simulink library "xpcnilib"  (Simulink 6.0)
settings: Solver=ode45  SolverMode=SingleTasking  StartTime=0.0  StopTime=10.0  RelTol=1e-3
undefined symbols (not defined in the file or in its folder): madnipcie, mctrnipcie, mctrnipciecap, mdacbisa, mdanipci670x, mdanipci671x, mdanipcie, mdionipci6527, mdionipcie, mencnipci660x, misa8255, mnigpib, mnipci660x, mpci8255
libraries: xpcmeasurementcomputinglib x6
(part 3 of 3)

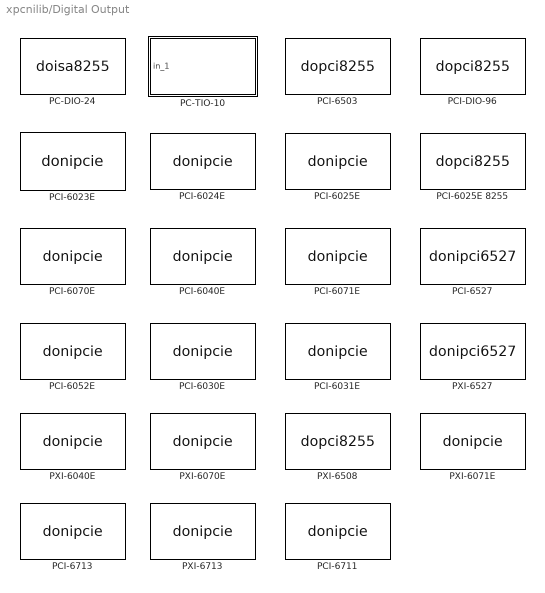
== system xpcnilib/Digital Output ==
  "PC-DIO-24 " : S-Function  InitFcn=misa8255(1);  FunctionName=doisa8255  Parameters=channel, port, reset, initValue, sampletime, baseaddress, control  mask(donipcdio24){channel=[1], port=A, reset=[1], initValue=[0], chip=1, sampletime=0.001, baseaddress=0x300}
      mask prompts: channel "Channel vector:"; reset "Reset vector:"; initValue "Initial value vector:"; sampletime "Sample time:"; baseaddress "Base address (i.e. 0xd000):"
      mask help:
      | PC-DIO-24
      | National Instruments
      | Digital Output
      mask init:
      | baseaddress=hex2dec(baseaddress(3:end));
      | control=155;
      | boardType=16;
      | [baseaddress,control,maskdisplay,maskdescription,reset,initValue]=misa8255(2, chip, port, channel, baseaddress, reset, initValue);
      | set_param(gcb, 'MaskDisplay', maskdisplay);
      | set_param(gcb, 'MaskDescription', maskdescription);
      mask Help: helpview(fullfile(docroot, 'mapfiles', 'xpc.map'), 'NationalInstruments_PC-DIO-24_DOUT')
      mask StyleString: edit,popup(A|B|C),edit,edit,popup(1),edit,edit
      mask Display: disp('PC-DIO-24\nNational Instr.\nDigital Output');port_label('input',1,'1');
  "PC-TIO-10 " : Subsystem  PropExecContextAcrossSSBoundary=on  mask(Digital Output Module){n_channels=1, port=PIA A, sample_time=0.001, baseaddress=0x300}
      mask prompts: n_channels "Number of channels:"; sample_time "Sample time:"; baseaddress "Base address (i.e. 0xd000):"
      mask help:
      | PC-TIO-10
      | National Instruments
      | Digital Output
      mask init:
      | baseaddress=hex2dec(baseaddress(3:end));
      mask Help: helpview(fullfile(docroot, 'mapfiles', 'xpc.map'), 'NationalInstruments_PC-TIO-10_DOUT')
      mask StyleString: edit,popup(PIA A|PIA B),edit,edit
      mask Display: disp('PC-TIO-10\nNational Instr.\nDigital Output')
  "PCI-6023E " : S-Function  InitFcn=mdionipcie(1);  FunctionName=donipcie  Parameters="channel,  reset, initValue, sampletime,slot, control, boardType"  mask(donipcie){channel=[1], reset=[1], initValue=[0], sampletime=0.001, slot=-1}
      mask prompts: channel "Channel vector:"; reset "Reset vector:"; initValue "Initial value vector:"; sampletime "Sample time:"; slot "PCI slot (-1: autosearch):"
      mask help:
      | PCI-6023E
      | National Instruments
      | Digital Output
      mask init:
      | control=0;
      | boardType=1;
      | [control,reset,initValue]=mdionipcie(2,channel,slot,2,boardType,reset,initValue);
      mask Help: helpview(fullfile(docroot, 'mapfiles', 'xpc.map'), 'NationalInstruments_PCI-6023E_DOUT')
      mask Display: disp('PCI-6023E\nNational Instr.\nDigital Output');port_label('input',1,'1');
  "PCI-6024E " : S-Function  InitFcn=mdionipcie(1);  FunctionName=donipcie  Parameters=channel, reset, initValue, sampletime,slot, control, boardType  mask(donipcie){channel=[1], reset=[1], initValue=[0], sampletime=0.001, slot=-1}
      mask prompts: channel "Channel vector:"; reset "Reset vector:"; initValue "Initial value vector:"; sampletime "Sample time:"; slot "PCI slot (-1: autosearch):"
      mask help:
      | PCI-6024E
      | National Instruments
      | Digital Output
      mask init:
      | control=0;
      | boardType=2;
      | [control,reset,initValue]=mdionipcie(2,channel,slot,2,boardType,reset,initValue);
      mask Help: helpview(fullfile(docroot, 'mapfiles', 'xpc.map'), 'NationalInstruments_PCI-6024E_DOUT')
      mask Display: disp('PCI-6024E\nNational Instr.\nDigital Output');port_label('input',1,'1');
  "PCI-6025E " : S-Function  InitFcn=mdionipcie(1);  FunctionName=donipcie  Parameters=channel, reset, initValue, sampletime,slot, control, boardType  mask(donipcie){channel=[1], reset=[1], initValue=[0], sampletime=0.001, slot=-1}
      mask prompts: channel "Channel vector:"; reset "Reset vector:"; initValue "Initial value vector:"; sampletime "Sample time:"; slot "PCI slot (-1: autosearch):"
      mask help:
      | PCI-6025E
      | National Instruments
      | Digital Output
      mask init:
      | control=0;
      | boardType=3;
      | [control,reset,initValue]=mdionipcie(2,channel,slot,2,boardType,reset,initValue);
      mask Help: helpview(fullfile(docroot, 'mapfiles', 'xpc.map'), 'NationalInstruments_PCI-6025E_DOUT')
      mask Display: disp('PCI-6025E\nNational Instr.\nDigital Output');port_label('input',1,'1');
  "PCI-6025E 8255 " : S-Function  InitFcn=mpci8255(1);  FunctionName=dopci8255  Parameters=channel, port, reset, initValue, chip, sampletime, slot, control, boardType  mask(donipci6025e8255){channel=[1], port=A, reset=[1], initValue=[0], chip=1, sampletime=0.001, slot=-1}
      mask prompts: channel "Channel vector:"; reset "Reset vector:"; initValue "Initial value vector:"; sampletime "Sample time:"; slot "PCI slot (-1: autosearch):"
      mask help:
      | PCI-6025E (8255)
      | National Instruments
      | Digital Output
      mask init:
      | control=155;
      | [boardType,control,maskdisplay,maskdescription, reset, initValue]=mpci8255(2, chip, port, channel, slot, reset, initValue);
      | set_param(gcb, 'MaskDisplay', maskdisplay);
      | set_param(gcb, 'MaskDescription', maskdescription);
      mask Help: helpview(fullfile(docroot, 'mapfiles', 'xpc.map'), 'NationalInstruments_PCI-6025E-8255_DOUT')
      mask StyleString: edit,popup(A|B|C),edit,edit,popup(1),edit,edit
      mask Display: disp('PCI-6025E (8255)\nNational Instr.\nDigital Output');port_label('input',1,'1');
  "PCI-6030E " : S-Function  InitFcn=mdionipcie(1);  FunctionName=donipcie  Parameters=channel, reset, initValue, sampletime,slot, control, boardType  mask(donipcie){channel=[1], reset=[1], initValue=[0], sampletime=0.001, slot=-1}
      mask prompts: channel "Channel vector:"; reset "Reset vector:"; initValue "Initial value vector:"; sampletime "Sample time:"; slot "PCI slot (-1: autosearch):"
      mask help:
      | PCI-6030E
      | National Instruments
      | Digital Output
      mask init:
      | control=0;
      | boardType=10;
      | [control,reset,initValue]=mdionipcie(2,channel,slot,2,boardType,reset,initValue);
      mask Help: helpview(fullfile(docroot, 'mapfiles', 'xpc.map'), 'NationalInstruments_PCI-MIO-16XE-10_DOUT')
      mask Display: disp('PCI-6030E\nNational Instr.\nDigital Output');port_label('input',1,'1');
  "PCI-6031E " : S-Function  InitFcn=mdionipcie(1);  FunctionName=donipcie  Parameters=channel, reset, initValue, sampletime,slot, control, boardType  mask(donipcie){channel=[1], reset=[1], initValue=[0], sampletime=0.001, slot=-1}
      mask prompts: channel "Channel vector:"; reset "Reset vector:"; initValue "Initial value vector:"; sampletime "Sample time:"; slot "PCI slot (-1: autosearch):"
      mask help:
      | PCI-6031E
      | National Instruments
      | Digital Output
      mask init:
      | control=0;
      | boardType=11;
      | [control,reset,initValue]=mdionipcie(2,channel,slot,2,boardType,reset,initValue);
      mask Help: helpview(fullfile(docroot, 'mapfiles', 'xpc.map'), 'NationalInstruments_PCI-6031E_DOUT')
      mask Display: disp('PCI-6031E\nNational Instr.\nDigital Output');port_label('input',1,'1');
  "PCI-6040E " : S-Function  InitFcn=mdionipcie(1);  FunctionName=donipcie  Parameters=channel, reset, initValue, sampletime,slot, control, boardType  mask(donipcie){channel=[1], reset=[1], initValue=[0], sampletime=0.001, slot=-1}
      mask prompts: channel "Channel vector:"; reset "Reset vector:"; initValue "Initial value vector:"; sampletime "Sample time:"; slot "PCI slot (-1: autosearch):"
      mask help:
      | PCI-6040E
      | National Instruments
      | Digital Output
      mask init:
      | control=0;
      | boardType=5;
      | [control,reset,initValue]=mdionipcie(2,channel,slot,2,boardType,reset,initValue);
      mask Help: helpview(fullfile(docroot, 'mapfiles', 'xpc.map'), 'NationalInstruments_PCI-MIO-16E-4_DOUT')
      mask Display: disp('PCI-6040E\nNational Instr.\nDigital Output');port_label('input',1,'1');
  "PCI-6052E " : S-Function  InitFcn=mdionipcie(1);  FunctionName=donipcie  Parameters=channel, reset, initValue, sampletime,slot, control, boardType  mask(donipcie){channel=[1], reset=[1], initValue=[0], sampletime=0.001, slot=-1}
      mask prompts: channel "Channel vector:"; reset "Reset vector:"; initValue "Initial value vector:"; sampletime "Sample time:"; slot "PCI slot (-1: autosearch):"
      mask help:
      | PCI-6052E
      | National Instruments
      | Digital Output
      mask init:
      | control=0;
      | boardType=9;
      | [control,reset,initValue]=mdionipcie(2,channel,slot,2,boardType,reset,initValue);
      mask Help: helpview(fullfile(docroot, 'mapfiles', 'xpc.map'), 'NationalInstruments_PCI-6052E_DOUT')
      mask Display: disp('PCI-6052E\nNational Instr.\nDigital Output');port_label('input',1,'1');
  "PCI-6070E " : S-Function  InitFcn=mdionipcie(1);  FunctionName=donipcie  Parameters=channel, reset, initValue, sampletime,slot, control, boardType  mask(donipcie){channel=[1], reset=[1], initValue=[0], sampletime=0.001, slot=-1}
      mask prompts: channel "Channel vector:"; reset "Reset vector:"; initValue "Initial value vector:"; sampletime "Sample time:"; slot "PCI slot (-1: autosearch):"
      mask help:
      | PCI-6070E
      | National Instruments
      | Digital Output
      mask init:
      | control=0;
      | boardType=4;
      | [control,reset,initValue]=mdionipcie(2,channel,slot,2,boardType,reset,initValue);
      mask Help: helpview(fullfile(docroot, 'mapfiles', 'xpc.map'), 'NationalInstruments_PCI-MIO-16E-1_DOUT')
      mask Display: disp('PCI-6070E\nNational Instr.\nDigital Output');port_label('input',1,'1');
  "PCI-6071E " : S-Function  InitFcn=mdionipcie(1);  FunctionName=donipcie  Parameters=channel, reset, initValue, sampletime,slot, control, boardType  mask(donipcie){channel=[1], reset=[1], initValue=[0], sampletime=0.001, slot=-1}
      mask prompts: channel "Channel vector:"; reset "Reset vector:"; initValue "Inital value vector:"; sampletime "Sample time:"; slot "PCI slot (-1: autosearch):"
      mask help:
      | PCI-6071E
      | National Instruments
      | Digital Output
      mask init:
      | control=0;
      | boardType=8;
      | [control,reset,initValue]=mdionipcie(2,channel,slot,2,boardType,reset,initValue);
      mask Help: helpview(fullfile(docroot, 'mapfiles', 'xpc.map'), 'NationalInstruments_PCI-6071E_DOUT')
      mask Display: disp('PCI-6071E\nNational Instr.\nDigital Output');port_label('input',1,'1');
  "PCI-6503 " : S-Function  InitFcn=mpci8255(1);  FunctionName=dopci8255  Parameters=channel, port, reset, initValue, chip, sampletime, slot, control, boardType  mask(donipci6503){channel=[1], port=A, reset=[1], initValue=[0], chip=1, sampletime=0.001, slot=-1}
      mask prompts: channel "Channel vector:"; reset "Reset vector:"; initValue "Initial value vector:"; sampletime "Sample time:"; slot "PCI slot (-1: autosearch):"
      mask help:
      | PCI-6503
      | National Instruments
      | Digital Output
      mask init: same as xpcnilib/Digital Output/PCI-6025E 8255 
      mask Help: helpview(fullfile(docroot, 'mapfiles', 'xpc.map'), 'NationalInstruments_PCI-6503_DOUT')
      mask StyleString: edit,popup(A|B|C),edit,edit,popup(1),edit,edit
      mask Display: disp('PCI-6503\nNational Instr.\nDigital Output');port_label('input',1,'1');
  "PCI-6527 " : S-Function  InitFcn=mdionipci6527(1);  FunctionName=donipci6527  Parameters=channel, port, reset, initValue, sample, slot,1  mask(donipci6527){channel=[1], port=A, reset=[1], initValue=[0], sample=0.001, slot=-1}
      mask prompts: channel "Channel vector:"; reset "Reset vector:"; initValue "Initial value vector:"; sample "Sample time:"; slot "PCI slot (-1: autosearch):"
      mask help:
      | PCI-6527
      | National Instruments
      | Digital Output
      mask init:
      | [filter, reset, initValue] = mdionipci6527( 2, channel, port, sample, slot, 2, 0, 0, reset, initValue );
      mask Help: helpview(fullfile(docroot, 'mapfiles', 'xpc.map'), 'NationalInstruments_PCI-6527_DOUT')
      mask StyleString: edit,popup(A|B|C),edit,edit,edit,edit
      mask Display: disp('PCI-6527\nNational Instr\nDigital Output');port_label('input',1,'1');
  "PCI-6711 " : S-Function  InitFcn=mdionipcie(1);  FunctionName=donipcie  Parameters="channel,  reset, initValue, sampletime,slot, control, boardType"  mask(donipcie){channel=[1], reset=[1], initValue=[0], sampletime=0.001, slot=-1}
      mask prompts: channel "Channel vector:"; reset "Reset vector:"; initValue "Initial value vector:"; sampletime "Sample time:"; slot "PCI slot (-1: autosearch):"
      mask help:
      | PCI-6711
      | National Instruments
      | Digital Output
      mask init:
      | control=0;
      | boardType=15;
      | [control,reset,initValue]=mdionipcie(2,channel,slot,2,boardType,reset,initValue);
      mask Help: helpview(fullfile(docroot, 'mapfiles', 'xpc.map'), 'NationalInstruments_PCI-6711_DOUT')
      mask Display: disp('PCI-6711 \nNational Instr.\nDigital Output');port_label('input',1,'1');
  "PCI-6713 " : S-Function  InitFcn=mdionipcie(1);  FunctionName=donipcie  Parameters="channel,  reset, initValue, sampletime,slot, control, boardType"  mask(donipcie){channel=[1], reset=[1], initValue=[0], sampletime=0.001, slot=-1}
      mask prompts: channel "Channel vector:"; reset "Reset vector:"; initValue "Initial value vector:"; sampletime "Sample time:"; slot "PCI slot (-1: autosearch):"
      mask help:
      | PCI-6713
      | National Instruments
      | Digital Output
      mask init:
      | control=0;
      | boardType=13;
      | [control,reset,initValue]=mdionipcie(2,channel,slot,2,boardType,reset,initValue);
      mask Help: helpview(fullfile(docroot, 'mapfiles', 'xpc.map'), 'NationalInstruments_PCI-6713_DOUT')
      mask Display: disp('PCI-6713 \nNational Instr.\nDigital Output');port_label('input',1,'1');
  "PCI-DIO-96 " : S-Function  InitFcn=mpci8255(1);  FunctionName=dopci8255  Parameters=channel, port, reset, initValue, chip, sampletime, slot, control, boardType  mask(donipcidio96){channel=[1], port=A, reset=[1], initValue=[0], chip=1, sampletime=0.001, slot=-1}
      mask prompts: channel "Channel vector:"; reset "Reset vector:"; initValue "Initial value vector:"; sampletime "Sample time:"; slot "PCI slot (-1: autosearch):"
      mask help:
      | PCI-DIO-96
      | National Instruments
      | Digital Output
      mask init: same as xpcnilib/Digital Output/PCI-6025E 8255 
      mask Help: helpview(fullfile(docroot, 'mapfiles', 'xpc.map'), 'NationalInstruments_PCI-DIO-96_DOUT')
      mask StyleString: edit,popup(A|B|C),edit,edit,popup(1|2|3|4),edit,edit
      mask Display: disp('PCI-DIO-96\nNational Instr.\nDigital Output');port_label('input',1,'1');
  "PXI-6040E " : S-Function  InitFcn=mdionipcie(1);  FunctionName=donipcie  Parameters=channel, reset, initValue, sampletime,slot, control, boardType  mask(donipcie){channel=[1], reset=[1], initValue=[0], sampletime=0.001, slot=-1}
      mask prompts: channel "Channel vector:"; reset "Reset vector:"; initValue "Initial value vector:"; sampletime "Sample time:"; slot "PCI slot (-1: autosearch):"
      mask help:
      | PXI-6040E
      | National Instruments
      | Digital Output
      mask init:
      | control=0;
      | boardType=7;
      | [control,reset,initValue]=mdionipcie(2,channel,slot,2,boardType,reset,initValue);
      mask Help: helpview(fullfile(docroot, 'mapfiles', 'xpc.map'), 'NationalInstruments_PXI-6040E_DOUT')
      mask Display: disp('PXI-6040E\nNational Instr.\nDigital Output');port_label('input',1,'1');
  "PXI-6070E " : S-Function  InitFcn=mdionipcie(1);  FunctionName=donipcie  Parameters=channel, reset, initValue, sampletime,slot, control, boardType  mask(donipcie){channel=[1], reset=[1], initValue=[0], sampletime=0.001, slot=-1}
      mask prompts: channel "Channel vector:"; reset "Reset vector:"; initValue "Initial value vector:"; sampletime "Sample time:"; slot "PCI slot (-1: autosearch):"
      mask help:
      | PXI-6070E
      | National Instruments
      | Digital Output
      mask init:
      | control=0;
      | boardType=6;
      | [control,reset,initValue]=mdionipcie(2,channel,slot,2,boardType,reset,initValue);
      mask Help: helpview(fullfile(docroot, 'mapfiles', 'xpc.map'), 'NationalInstruments_PXI-6070E_DOUT')
      mask Display: disp('PXI-6070E\nNational Instr.\nDigital Output');port_label('input',1,'1');
  "PXI-6071E " : S-Function  InitFcn=mdionipcie(1);  FunctionName=donipcie  Parameters=channel, reset, initValue, sampletime,slot, control, boardType  mask(donipcie){channel=[1], reset=[1], initValue=[0], sampletime=0.001, slot=-1}
      mask prompts: channel "Channel vector:"; reset "Reset vector:"; initValue "Inital value vector:"; sampletime "Sample time:"; slot "PCI slot (-1: autosearch):"
      mask help:
      | PXI-6071E
      | National Instruments
      | Digital Output
      mask init:
      | control=0;
      | boardType=12;
      | [control,reset,initValue]=mdionipcie(2,channel,slot,2,boardType,reset,initValue);
      mask Help: helpview(fullfile(docroot, 'mapfiles', 'xpc.map'), 'NationalInstruments_PXI-6071E_DOUT')
      mask Display: disp('PXI-6071E\nNational Instr.\nDigital Output');port_label('input',1,'1');
  "PXI-6508 " : S-Function  InitFcn=mpci8255(1);  FunctionName=dopci8255  Parameters=channel, port, reset, initValue, chip, sampletime, slot, control, boardType  mask(donipxi6508){channel=[1], port=A, reset=[1], initValue=[0], chip=1, sampletime=0.001, slot=-1}
      mask prompts: channel "Channel vector:"; reset "Reset vector:"; initValue "Initial value vector:"; sampletime "Sample time:"; slot "PCI slot (-1: autosearch):"
      mask help:
      | PXI-6508
      | National Instruments
      | Digital Output
      mask init: same as xpcnilib/Digital Output/PCI-6025E 8255 
      mask Help: helpview(fullfile(docroot, 'mapfiles', 'xpc.map'), 'NationalInstruments_PXI-6508_DOUT')
      mask StyleString: edit,popup(A|B|C),edit,edit,popup(1|2|3|4),edit,edit
      mask Display: disp('PXI-6508\nNational Instr.\nDigital Output');port_label('input',1,'1');
  "PXI-6527 " : S-Function  InitFcn=mdionipci6527(1);  FunctionName=donipci6527  Parameters=channel, port, reset, initValue, sample, slot,2  mask(donipxi6527){channel=[1], port=A, reset=[1], initValue=[0], sample=-1, slot=-1}
      mask prompts: channel "Channel vector:"; reset "Reset vector:"; initValue "Initial value vector:"; sample "Sample time:"; slot "PCI slot (-1: autosearch):"
      mask help:
      | PXI-6527
      | National Instruments
      | Digital Output
      mask init:
      | [filter, reset, initValue] = mdionipci6527( 2, channel, port, sample, slot, 2, 0, 0, reset, initValue );
      mask Help: helpview(fullfile(docroot, 'mapfiles', 'xpc.map'), 'NationalInstruments_PXI-6527_DOUT')
      mask StyleString: edit,popup(A|B|C),edit,edit,edit,edit
      mask Display: disp('PXI-6527\nNational Instr\nDigital Output');port_label('input',1,'1');
  "PXI-6713 " : S-Function  InitFcn=mdionipcie(1);  FunctionName=donipcie  Parameters="channel,  reset, initValue, sampletime,slot, control, boardType"  mask(donipcie){channel=[1], reset=[1], initValue=[0], sampletime=0.001, slot=-1}
      mask prompts: channel "Channel vector:"; reset "Reset vector:"; initValue "Initial value vector:"; sampletime "Sample time:"; slot "PCI slot (-1: autosearch):"
      mask help:
      | PXI-6713
      | National Instruments
      | Digital Output
      mask init:
      | control=0;
      | boardType=14;
      | [control,reset,initValue]=mdionipcie(2,channel,slot,2,boardType,reset,initValue);
      mask Help: helpview(fullfile(docroot, 'mapfiles', 'xpc.map'), 'NationalInstruments_PXI-6713_DOUT')
      mask Display: disp('PXI-6713 \nNational Instr.\nDigital Output');port_label('input',1,'1');

== system xpcnilib/GPIB ==
  "GPIB-232CT-A " : S-Function  InitFcn=mnigpib(0);  FunctionName=rs232setup  Parameters=port, baud, dbits, sbits, parity, prot, sbuf, rbuf, 0, istr, iack, iackto, tstr, tack, tackto, initinfo, initackinfo, terminfo, termackinfo  mask(rs232setup){gpibid=0, port=COM1, baud=38400, dbits=8, sbits=1, parity=None, prot=None, sbuf=1024, rbuf=1024, initstr=[], termstr=[]}
      mask prompts: gpibid "GPIB address:"; baud "Baud rate:"; dbits "Number of data bits:"; sbits "Number of stop bits:"; prot "Protocol:"; sbuf "Send buffer size:"; rbuf "Receive buffer size:"; initstr "Initialization command structure:"; termstr "Termination command structure:"
      mask help:
      | GPIB-232CT-A
      | National Instruments
      | Setup
      mask init:
      | dmy = '';
      | [istr,iack,dmy,maskdisplay,maskdescription,dmy,dmy,dmy,dmy,initinfo,initackinfo,iackto]=mnigpib(2,initstr,4, gpibid);
      | [tstr,tack,dmy,maskdisplay,maskdescription,dmy,dmy,dmy,dmy,terminfo,termackinfo,tackto]=mnigpib(1,termstr,4, -gpibid);
      | set_param(gcb,'MaskDisplay',maskdisplay);
      | set_param(gcb,'MaskDescription',maskdescription);
      mask Help: helpview(fullfile(docroot, 'mapfiles', 'xpc.map'), 'NationalInstruments_GPIB-232CT-A_GPIB')
      mask StyleString: edit,popup(COM1|COM2|COM3|COM4),popup(115200|57600|38400|19200|9600|4800|2400|1200|600|300|110),popup(8|7),popup(1|2),popup(None|Odd|Even),popup(None|XOn XOff),edit,edit,edit,edit
      mask Display: disp('GPIB-232CT-A\nNational Instruments\nSetup');
  GPIB-232CT-A 1 : S-Function  FunctionName=rs232sendrec  Parameters=port, inStr, outStr, inport, outport, numinports, numoutports, formatsendinfo, formatrecinfo, waitarg, dtypes, ts, numeom, timeout  mask(rs232sendrec){port=COM1, blockvar=[], ts=0.1}
      mask prompts: blockvar "Message structure:"; ts "Sample time:"
      mask help:
      | GPIB-232CT-A
      | National Instruments
      | Send/Receive
      mask init:
      | inStr = '';
      | outStr = '';
      | [inStr,outStr,dtypes,maskdisplay,maskdescription,inport,outport, numinports, numoutports, formatsendinfo, formatrecinfo, waitarg, numeom, timeout] = mnigpib (1, blockvar, 3, -1);
      | set_param(gcb,'MaskDisplay',maskdisplay);
      | set_param(gcb,'MaskDescription',maskdescription);
      mask Help: helpview(fullfile(docroot, 'mapfiles', 'xpc.map'), 'NationalInstruments_GPIB-232CT-A-1_GPIB')
      mask StyleString: popup(COM1|COM2|COM3|COM4),edit,edit
      mask Display: disp('GPIB-232CT-A\nNational Instruments\nSend/Receive');

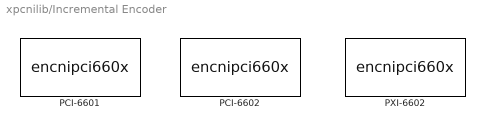
== system xpcnilib/Incremental Encoder ==
  "PCI-6601 " : S-Function  InitFcn=mencnipci660x(1);  FunctionName=encnipci660x  Parameters=device, channel, countMode, initCount, reload, indexPhase, filter, sampleTime, pciBus, pciSlot  mask(encnipci6601){channel=1, countMode=Quadrature Mode X4, initCount=0, reload=off, indexPhase=A low B low, filter=None, sampleTime=0.001, slot=-1}
      mask prompts: countMode "Counting mode:"; initCount "Initial count:"; reload "Reload at index pulse"; indexPhase "Index phase:"; sampleTime "Sample time:"; slot "PCI slot (-1: autosearch):"
      mask help:
      | PCI-6601
      | National Instr.
      | Inc. Encoder
      mask init:
      | phase = 2;
      | device = 0;
      | [maskDisplay, maskDescription, pciBus, pciSlot] = ...
      | 	mencnipci660x( phase, device, channel, initCount, slot );
      | set_param(gcb, 'MaskDisplay', maskDisplay);
      | set_param(gcb, 'MaskDescription', maskDescription);
      mask Help: helpview(fullfile(docroot, 'mapfiles', 'xpc.map'), 'NI_PCI-6601_Encoder')
      mask StyleString: popup(1|2|3|4),popup(Normal|Quadrature Mode X1|Quadrature Mode X2|Quadrature Mode X4|Two-pulse mode|Synchronous Source Mode),edit,checkbox,popup(A low B low|A low B high|A high B low|A high B high),popup(None|Synchronize input  to Timebase 3 (80MHz)|Minimum pulse width 5 microsec|Minimum pulse width 1 microsec|Minimum pulse width 500 nanosec|Minimum pulse width 100 nanosec|Minimum pulse width 25 nanosec),edit,edit
      mask Display: disp('PCI-6601\nNational Instr.\nInc. Encoder'); port_label('output', 1, '1');
  "PCI-6602 " : S-Function  InitFcn=mencnipci660x(1);  FunctionName=encnipci660x  Parameters=device, channel, countMode, initCount, reload, indexPhase, filter, sampleTime, pciBus, pciSlot  mask(encnipci6602){channel=1, countMode=Quadrature Mode X4, initCount=0, reload=off, indexPhase=A low B low, filter=None, sampleTime=0.001, slot=-1}
      mask prompts: countMode "Counting mode:"; initCount "Initial count:"; reload "Reload at index pulse"; indexPhase "Index phase:"; sampleTime "Sample time:"; slot "PCI slot (-1: autosearch):"
      mask help:
      | PCI-6602
      | National Instr.
      | Inc. Encoder
      mask init:
      | phase = 2;
      | device = 1;
      | [maskDisplay, maskDescription, pciBus, pciSlot] = ...
      | 	mencnipci660x( phase, device, channel, initCount, slot );
      | set_param(gcb, 'MaskDisplay', maskDisplay);
      | set_param(gcb, 'MaskDescription', maskDescription);
      mask Help: helpview(fullfile(docroot, 'mapfiles', 'xpc.map'), 'NI_PCI-6602_Encoder')
      mask StyleString: popup(1|2|3|4|5|6|7|8),popup(Normal|Quadrature Mode X1|Quadrature Mode X2|Quadrature Mode X4|Two-pulse mode|Synchronous Source Mode),edit,checkbox,popup(A low B low|A low B high|A high B low|A high B high),popup(None|Synchronize input  to Timebase 3 (80MHz)|Minimum pulse width 5 microsec|Minimum pulse width 1 microsec|Minimum pulse width 500 nanosec|Minimum pulse width 100 nanosec|Minimum pulse width 25 nanosec),edit,edit
      mask Display: disp('PCI-6602\nNational Instr.\nInc. Encoder'); port_label('output', 1, '1');
  "PXI-6602 " : S-Function  InitFcn=mencnipci660x(1);  FunctionName=encnipci660x  Parameters=device, channel, countMode, initCount, reload, indexPhase, filter, sampleTime, pciBus, pciSlot  mask(encnipxi6602){channel=1, countMode=Quadrature Mode X4, initCount=0, reload=off, indexPhase=A low B low, filter=None, sampleTime=0.001, slot=-1}
      mask prompts: countMode "Counting mode:"; initCount "Initial count:"; reload "Reload at index pulse"; indexPhase "Index phase:"; sampleTime "Sample time:"; slot "PCI slot (-1: autosearch):"
      mask help:
      | PXI-6602
      | National Instr.
      | Inc. Encoder
      mask init:
      | phase = 2;
      | device = 2;
      | [maskDisplay, maskDescription, pciBus, pciSlot] = mencnipci660x( phase, device, channel, initCount, slot );
      | set_param(gcb, 'MaskDisplay', maskDisplay);
      | set_param(gcb, 'MaskDescription', maskDescription);
      mask Help: helpview(fullfile(docroot, 'mapfiles', 'xpc.map'), 'NI_PXI-6602_Encoder')
      mask StyleString: popup(1|2|3|4|5|6|7|8),popup(Normal|Quadrature Mode X1|Quadrature Mode X2|Quadrature Mode X4|Synchronous Source Mode|Two-pulse mode),edit,checkbox,popup(A low B low|A low B high|A high B low|A high B high),popup(None|Synchronize input  to Timebase 3 (80MHz)|Minimum pulse width 5 microsec|Minimum pulse width 1 microsec|Minimum pulse width 500 nanosec|Minimum pulse width 100 nanosec|Minimum pulse width 25 nanosec),edit,edit
      mask Display: disp('PXI-6602\nNational Instr.\nInc. Encoder'); port_label('output', 1, '1');

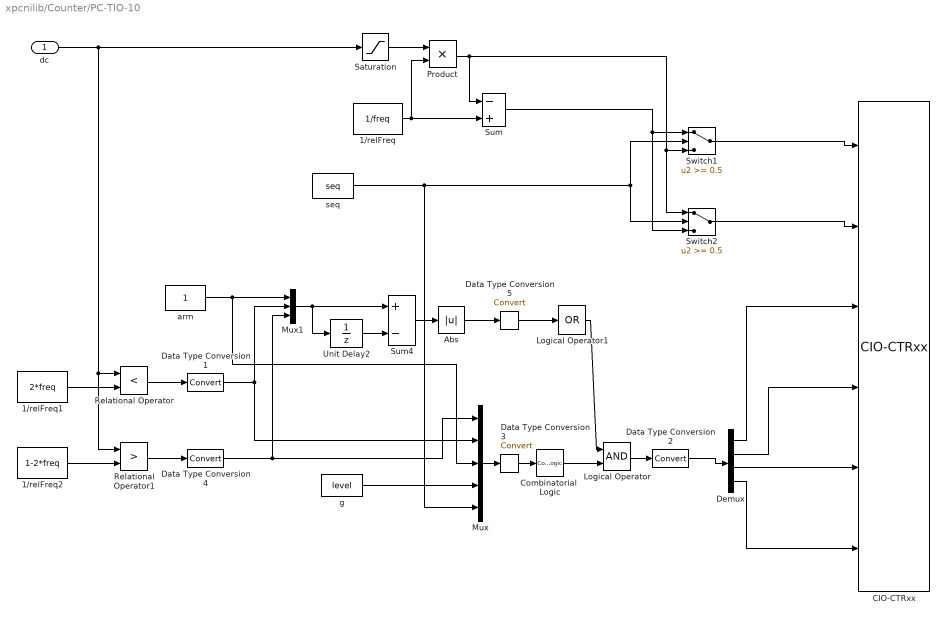
== system xpcnilib/Counter/PC-TIO-10  ==
  dc : Inport  LatchInput=off
  1/relFreq : Constant  Value=1/freq
  1/relFreq1 : Constant  Value=2*freq
  1/relFreq2 : Constant  Value=1-2*freq
  Abs : Abs  SaturateOnIntegerOverflow=on
  "CIO-CTRxx " : xpcmeasurementcomputinglib/Counter/CIO-CTRxx   mastermode=MasterMode  countermode=CounterMode  init=Init  commands=Runtime  term=Term  ts=Ts  baseAddress=baseAddress
  Combinatorial  Logic : CombinatorialLogic  TruthTable=[0,0,1,0;0,0,1,0;0,0,0,1;0,0,0,1;0,1,0,0;1,0,0,0;0,1,0,0;1,0,0,0;0,0,1,0;0,0,1,0;0,0,0,1;0,0,0,1;0,0,1,0;0,0,1,0;0,0,1,0;0,0,1,0;0,0,1,0;0,0,1,0;0,0,0,1;0,0,0,1;0,0,0,1;0,0,0,1;0,0,0,1;0,0,0,1;0,0,0,0;0,0,0,0;0,0,0,0;0,0,0,0;0,0,0,0;0,0,0,0;0,0,0,0;0,0,0,0]
  Data Type Conversion1 : DataTypeConversion  OutDataTypeMode=double  SaturateOnIntegerOverflow=on  RndMeth=Zero
  Data Type Conversion2 : DataTypeConversion  SaturateOnIntegerOverflow=on  RndMeth=Zero
  Data Type Conversion3 : DataTypeConversion  SaturateOnIntegerOverflow=on  RndMeth=Zero
  Data Type Conversion4 : DataTypeConversion  OutDataTypeMode=double  SaturateOnIntegerOverflow=on  RndMeth=Zero
  Data Type Conversion5 : DataTypeConversion  SaturateOnIntegerOverflow=on  RndMeth=Zero
  Demux : Demux
  Logical Operator : Logic
  Logical Operator1 : Logic  Operator=OR  Inputs=1
  Mux : Mux  Inputs=5
  Mux1 : Mux  Inputs=3
  Product : Product  SaturateOnIntegerOverflow=on  InputSameDT=on
  Relational Operator : RelationalOperator  Operator=<  InputSameDT=on
  Relational Operator1 : RelationalOperator  Operator=>  InputSameDT=on
  Saturation : Saturate  UpperLimit=1-2*freq  LowerLimit=2*freq  ZeroCross=off
  Sum : Sum  Inputs=-+  SaturateOnIntegerOverflow=on  InputSameDT=on
  Sum4 : Sum  Inputs=+-  SaturateOnIntegerOverflow=on  InputSameDT=on
  Switch1 : Switch  Threshold=0.5  InputSameDT=on
  Switch2 : Switch  Threshold=0.5  InputSameDT=on
  Unit Delay2 : UnitDelay  X0=2  SampleTime=Ts
  arm : Constant
  g : Constant  Value=level
  seq : Constant  Value=seq
  wires:
  Data Type Conversion5/1 -> Logical Operator1/1
  Data Type Conversion3/1 -> Combinatorial  Logic/1
  Data Type Conversion2/1 -> Demux/1
  Data Type Conversion1/1 -> Mux/2, Mux1/2
  Data Type Conversion4/1 -> Mux/1, Mux1/3
  Switch2/1 -> "CIO-CTRxx "/2
  Switch1/1 -> "CIO-CTRxx "/1
  Mux/1 -> Data Type Conversion3/1
  Abs/1 -> Data Type Conversion5/1
  arm/1 -> Mux/3, Mux1/1
  Mux1/1 -> Unit Delay2/1, Sum4/1
  dc/1 -> Relational Operator1/1, Relational Operator/1, Saturation/1
  Saturation/1 -> Product/1
  Sum/1 -> Switch2/3, Switch1/1
  seq/1 -> Mux/5, Switch2/2, Switch1/2
  g/1 -> Mux/4
  Demux/4 -> "CIO-CTRxx "/6
  Demux/3 -> "CIO-CTRxx "/5
  Demux/2 -> "CIO-CTRxx "/4
  Demux/1 -> "CIO-CTRxx "/3
  Logical Operator1/1 -> Logical Operator/1
  Sum4/1 -> Abs/1
  Unit Delay2/1 -> Sum4/2
  Logical Operator/1 -> Data Type Conversion2/1
  Combinatorial  Logic/1 -> Logical Operator/2
  Relational Operator/1 -> Data Type Conversion1/1
  Relational Operator1/1 -> Data Type Conversion4/1
  1/relFreq2/1 -> Relational Operator1/2
  Product/1 -> Switch2/1, Switch1/3, Sum/1
  1/relFreq/1 -> Sum/2, Product/2
  1/relFreq1/1 -> Relational Operator/2

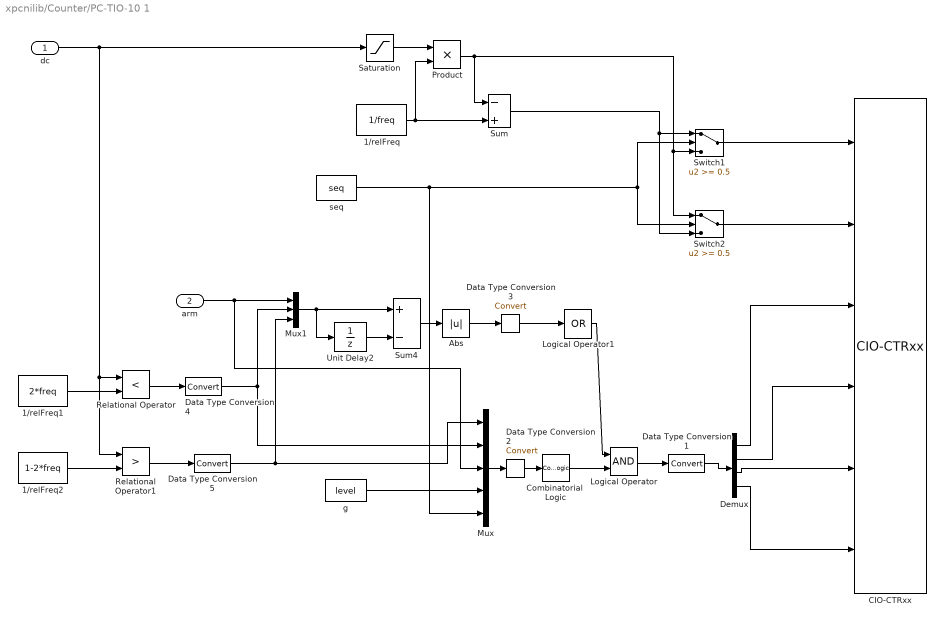
== system xpcnilib/Counter/PC-TIO-10 1 ==
  dc : Inport  LatchInput=off
  arm : Inport  Port=2  LatchInput=off
  1/relFreq : Constant  Value=1/freq
  1/relFreq1 : Constant  Value=2*freq
  1/relFreq2 : Constant  Value=1-2*freq
  Abs : Abs  SaturateOnIntegerOverflow=on
  "CIO-CTRxx " : xpcmeasurementcomputinglib/Counter/CIO-CTRxx   mastermode=MasterMode  countermode=CounterMode  init=Init  commands=Runtime  term=Term  ts=Ts  baseAddress=baseAddress
  Combinatorial  Logic : CombinatorialLogic  TruthTable=[0,0,1,0;0,0,1,0;0,0,0,1;0,0,0,1;0,1,0,0;1,0,0,0;0,1,0,0;1,0,0,0;0,0,1,0;0,0,1,0;0,0,0,1;0,0,0,1;0,0,1,0;0,0,1,0;0,0,1,0;0,0,1,0;0,0,1,0;0,0,1,0;0,0,0,1;0,0,0,1;0,0,0,1;0,0,0,1;0,0,0,1;0,0,0,1;0,0,0,0;0,0,0,0;0,0,0,0;0,0,0,0;0,0,0,0;0,0,0,0;0,0,0,0;0,0,0,0]
  Data Type Conversion1 : DataTypeConversion  SaturateOnIntegerOverflow=on  RndMeth=Zero
  Data Type Conversion2 : DataTypeConversion  SaturateOnIntegerOverflow=on  RndMeth=Zero
  Data Type Conversion3 : DataTypeConversion  SaturateOnIntegerOverflow=on  RndMeth=Zero
  Data Type Conversion4 : DataTypeConversion  OutDataTypeMode=double  SaturateOnIntegerOverflow=on  RndMeth=Zero
  Data Type Conversion5 : DataTypeConversion  OutDataTypeMode=double  SaturateOnIntegerOverflow=on  RndMeth=Zero
  Demux : Demux
  Logical Operator : Logic
  Logical Operator1 : Logic  Operator=OR  Inputs=1
  Mux : Mux  Inputs=5
  Mux1 : Mux  Inputs=3
  Product : Product  SaturateOnIntegerOverflow=on  InputSameDT=on
  Relational Operator : RelationalOperator  Operator=<  InputSameDT=on
  Relational Operator1 : RelationalOperator  Operator=>  InputSameDT=on
  Saturation : Saturate  UpperLimit=1-2*freq  LowerLimit=2*freq  ZeroCross=off
  Sum : Sum  Inputs=-+  SaturateOnIntegerOverflow=on  InputSameDT=on
  Sum4 : Sum  Inputs=+-  SaturateOnIntegerOverflow=on  InputSameDT=on
  Switch1 : Switch  Threshold=0.5  InputSameDT=on
  Switch2 : Switch  Threshold=0.5  InputSameDT=on
  Unit Delay2 : UnitDelay  X0=2  SampleTime=Ts
  g : Constant  Value=level
  seq : Constant  Value=seq
  wires:
  Data Type Conversion5/1 -> Mux/1, Mux1/3
  Data Type Conversion4/1 -> Mux/2, Mux1/2
  Data Type Conversion3/1 -> Logical Operator1/1
  Data Type Conversion2/1 -> Combinatorial  Logic/1
  Data Type Conversion1/1 -> Demux/1
  Switch2/1 -> "CIO-CTRxx "/2
  Switch1/1 -> "CIO-CTRxx "/1
  Mux/1 -> Data Type Conversion2/1
  Abs/1 -> Data Type Conversion3/1
  arm/1 -> Mux/3, Mux1/1
  Mux1/1 -> Unit Delay2/1, Sum4/1
  dc/1 -> Relational Operator1/1, Relational Operator/1, Saturation/1
  Saturation/1 -> Product/1
  Sum/1 -> Switch2/3, Switch1/1
  seq/1 -> Mux/5, Switch2/2, Switch1/2
  g/1 -> Mux/4
  Demux/4 -> "CIO-CTRxx "/6
  Demux/3 -> "CIO-CTRxx "/5
  Demux/2 -> "CIO-CTRxx "/4
  Demux/1 -> "CIO-CTRxx "/3
  Logical Operator1/1 -> Logical Operator/1
  Sum4/1 -> Abs/1
  Unit Delay2/1 -> Sum4/2
  Logical Operator/1 -> Data Type Conversion1/1
  Combinatorial  Logic/1 -> Logical Operator/2
  Relational Operator/1 -> Data Type Conversion4/1
  Relational Operator1/1 -> Data Type Conversion5/1
  1/relFreq2/1 -> Relational Operator1/2
  Product/1 -> Switch2/1, Switch1/3, Sum/1
  1/relFreq/1 -> Sum/2, Product/2
  1/relFreq1/1 -> Relational Operator/2

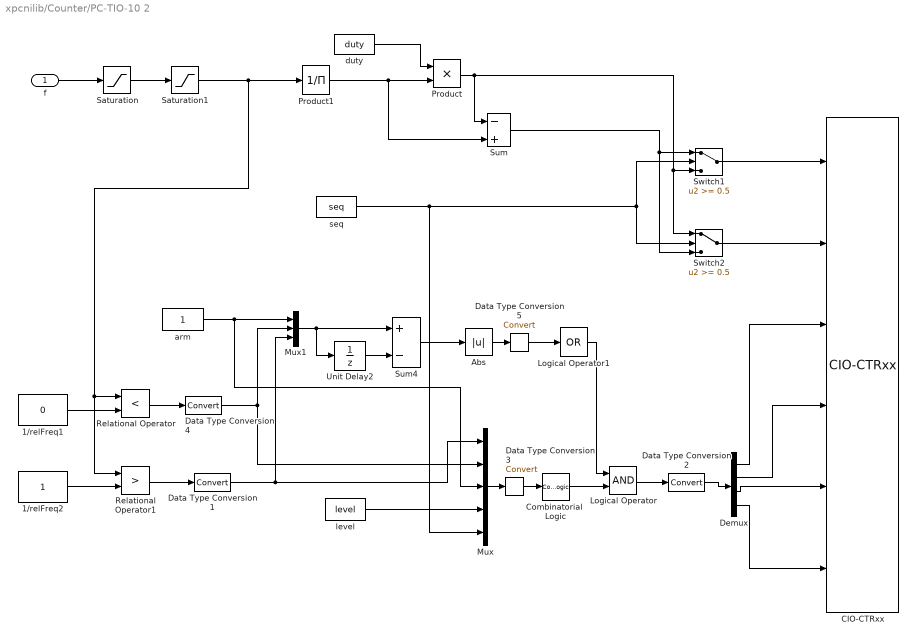
== system xpcnilib/Counter/PC-TIO-10 2 ==
  f : Inport  LatchInput=off
  1/relFreq1 : Constant  Value=0
  1/relFreq2 : Constant
  Abs : Abs  SaturateOnIntegerOverflow=on
  "CIO-CTRxx " : xpcmeasurementcomputinglib/Counter/CIO-CTRxx   mastermode=MasterMode  countermode=CounterMode  init=Init  commands=Runtime  term=Term  ts=Ts  baseAddress=baseAddress
  Combinatorial  Logic : CombinatorialLogic  TruthTable=[0,0,1,0;0,0,1,0;0,0,0,1;0,0,0,1;0,1,0,0;1,0,0,0;0,1,0,0;1,0,0,0;0,0,1,0;0,0,1,0;0,0,0,1;0,0,0,1;0,0,1,0;0,0,1,0;0,0,1,0;0,0,1,0;0,0,1,0;0,0,1,0;0,0,0,1;0,0,0,1;0,0,0,1;0,0,0,1;0,0,0,1;0,0,0,1;0,0,0,0;0,0,0,0;0,0,0,0;0,0,0,0;0,0,0,0;0,0,0,0;0,0,0,0;0,0,0,0]
  Data Type Conversion1 : DataTypeConversion  OutDataTypeMode=double  SaturateOnIntegerOverflow=on  RndMeth=Zero
  Data Type Conversion2 : DataTypeConversion  SaturateOnIntegerOverflow=on  RndMeth=Zero
  Data Type Conversion3 : DataTypeConversion  SaturateOnIntegerOverflow=on  RndMeth=Zero
  Data Type Conversion4 : DataTypeConversion  OutDataTypeMode=double  SaturateOnIntegerOverflow=on  RndMeth=Zero
  Data Type Conversion5 : DataTypeConversion  SaturateOnIntegerOverflow=on  RndMeth=Zero
  Demux : Demux
  Logical Operator : Logic
  Logical Operator1 : Logic  Operator=OR  Inputs=1
  Mux : Mux  Inputs=5
  Mux1 : Mux  Inputs=3
  Product : Product  SaturateOnIntegerOverflow=on  InputSameDT=on
  Product1 : Product  Inputs=/  SaturateOnIntegerOverflow=on  InputSameDT=on
  Relational Operator : RelationalOperator  Operator=<  InputSameDT=on
  Relational Operator1 : RelationalOperator  Operator=>  InputSameDT=on
  Saturation : Saturate  UpperLimit=duty/2  LowerLimit=duty/(2^16-1)  ZeroCross=off
  Saturation1 : Saturate  UpperLimit=(1-duty)/2  LowerLimit=(1-duty)/(2^16-1)  ZeroCross=off
  Sum : Sum  Inputs=-+  SaturateOnIntegerOverflow=on  InputSameDT=on
  Sum4 : Sum  Inputs=+-  SaturateOnIntegerOverflow=on  InputSameDT=on
  Switch1 : Switch  Threshold=0.5  InputSameDT=on
  Switch2 : Switch  Threshold=0.5  InputSameDT=on
  Unit Delay2 : UnitDelay  X0=2  SampleTime=Ts
  arm : Constant
  duty : Constant  Value=duty
  level : Constant  Value=level
  seq : Constant  Value=seq
  wires:
  Data Type Conversion5/1 -> Logical Operator1/1
  Data Type Conversion3/1 -> Combinatorial  Logic/1
  Data Type Conversion2/1 -> Demux/1
  Data Type Conversion1/1 -> Mux/1, Mux1/3
  Data Type Conversion4/1 -> Mux/2, Mux1/2
  Product1/1 -> Sum/2, Product/2
  duty/1 -> Product/1
  Saturation1/1 -> Relational Operator/1, Relational Operator1/1, Product1/1
  Mux/1 -> Data Type Conversion3/1
  Abs/1 -> Data Type Conversion5/1
  arm/1 -> Mux/3, Mux1/1
  Mux1/1 -> Unit Delay2/1, Sum4/1
  f/1 -> Saturation/1
  Saturation/1 -> Saturation1/1
  Sum/1 -> Switch2/3, Switch1/1
  seq/1 -> Mux/5, Switch2/2, Switch1/2
  Switch2/1 -> "CIO-CTRxx "/2
  Switch1/1 -> "CIO-CTRxx "/1
  level/1 -> Mux/4
  Demux/4 -> "CIO-CTRxx "/6
  Demux/3 -> "CIO-CTRxx "/5
  Demux/2 -> "CIO-CTRxx "/4
  Demux/1 -> "CIO-CTRxx "/3
  Logical Operator1/1 -> Logical Operator/1
  Sum4/1 -> Abs/1
  Unit Delay2/1 -> Sum4/2
  Logical Operator/1 -> Data Type Conversion2/1
  Combinatorial  Logic/1 -> Logical Operator/2
  Relational Operator/1 -> Data Type Conversion4/1
  Relational Operator1/1 -> Data Type Conversion1/1
  1/relFreq2/1 -> Relational Operator1/2
  Product/1 -> Switch2/1, Switch1/3, Sum/1
  1/relFreq1/1 -> Relational Operator/2

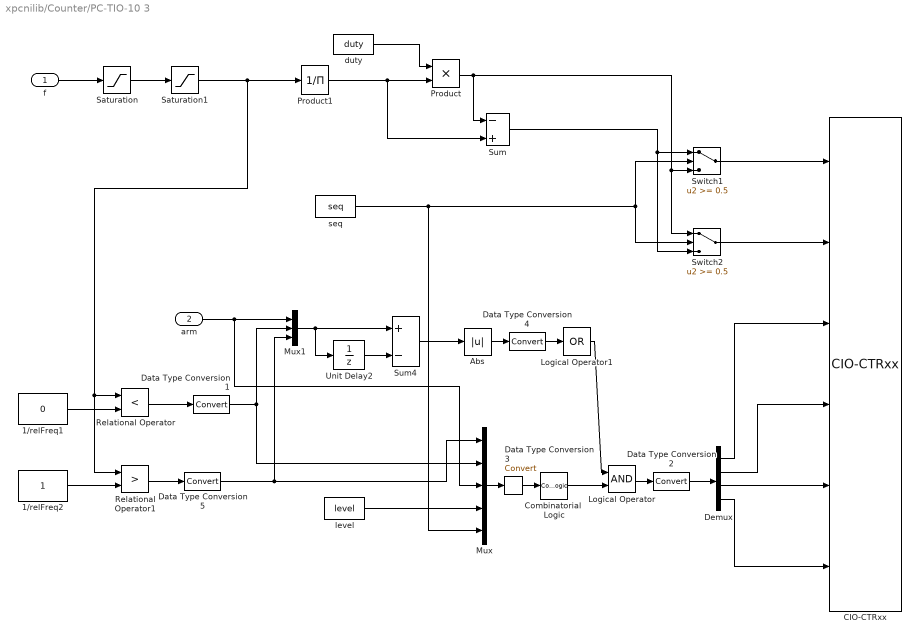
== system xpcnilib/Counter/PC-TIO-10 3 ==
  f : Inport  LatchInput=off
  arm : Inport  Port=2  LatchInput=off
  1/relFreq1 : Constant  Value=0
  1/relFreq2 : Constant
  Abs : Abs  SaturateOnIntegerOverflow=on
  "CIO-CTRxx " : xpcmeasurementcomputinglib/Counter/CIO-CTRxx   mastermode=MasterMode  countermode=CounterMode  init=Init  commands=Runtime  term=Term  ts=Ts  baseAddress=baseAddress
  Combinatorial  Logic : CombinatorialLogic  TruthTable=[0,0,1,0;0,0,1,0;0,0,0,1;0,0,0,1;0,1,0,0;1,0,0,0;0,1,0,0;1,0,0,0;0,0,1,0;0,0,1,0;0,0,0,1;0,0,0,1;0,0,1,0;0,0,1,0;0,0,1,0;0,0,1,0;0,0,1,0;0,0,1,0;0,0,0,1;0,0,0,1;0,0,0,1;0,0,0,1;0,0,0,1;0,0,0,1;0,0,0,0;0,0,0,0;0,0,0,0;0,0,0,0;0,0,0,0;0,0,0,0;0,0,0,0;0,0,0,0]
  Data Type Conversion1 : DataTypeConversion  OutDataTypeMode=double  SaturateOnIntegerOverflow=on  RndMeth=Zero
  Data Type Conversion2 : DataTypeConversion  SaturateOnIntegerOverflow=on  RndMeth=Zero
  Data Type Conversion3 : DataTypeConversion  SaturateOnIntegerOverflow=on  RndMeth=Zero
  Data Type Conversion4 : DataTypeConversion  SaturateOnIntegerOverflow=on  RndMeth=Zero
  Data Type Conversion5 : DataTypeConversion  OutDataTypeMode=double  SaturateOnIntegerOverflow=on  RndMeth=Zero
  Demux : Demux
  Logical Operator : Logic
  Logical Operator1 : Logic  Operator=OR  Inputs=1
  Mux : Mux  Inputs=5
  Mux1 : Mux  Inputs=3
  Product : Product  SaturateOnIntegerOverflow=on  InputSameDT=on
  Product1 : Product  Inputs=/  SaturateOnIntegerOverflow=on  InputSameDT=on
  Relational Operator : RelationalOperator  Operator=<  InputSameDT=on
  Relational Operator1 : RelationalOperator  Operator=>  InputSameDT=on
  Saturation : Saturate  UpperLimit=duty/2  LowerLimit=duty/(2^16-1)  ZeroCross=off
  Saturation1 : Saturate  UpperLimit=(1-duty)/2  LowerLimit=(1-duty)/(2^16-1)  ZeroCross=off
  Sum : Sum  Inputs=-+  SaturateOnIntegerOverflow=on  InputSameDT=on
  Sum4 : Sum  Inputs=+-  SaturateOnIntegerOverflow=on  InputSameDT=on
  Switch1 : Switch  Threshold=0.5  InputSameDT=on
  Switch2 : Switch  Threshold=0.5  InputSameDT=on
  Unit Delay2 : UnitDelay  X0=2  SampleTime=Ts
  duty : Constant  Value=duty
  level : Constant  Value=level
  seq : Constant  Value=seq
  wires:
  Data Type Conversion5/1 -> Mux/1, Mux1/3
  Data Type Conversion1/1 -> Mux/2, Mux1/2
  Data Type Conversion4/1 -> Logical Operator1/1
  Data Type Conversion3/1 -> Combinatorial  Logic/1
  Data Type Conversion2/1 -> Demux/1
  Product1/1 -> Sum/2, Product/2
  duty/1 -> Product/1
  Saturation1/1 -> Relational Operator/1, Relational Operator1/1, Product1/1
  Mux/1 -> Data Type Conversion3/1
  Abs/1 -> Data Type Conversion4/1
  arm/1 -> Mux/3, Mux1/1
  Mux1/1 -> Unit Delay2/1, Sum4/1
  f/1 -> Saturation/1
  Saturation/1 -> Saturation1/1
  Sum/1 -> Switch2/3, Switch1/1
  seq/1 -> Mux/5, Switch2/2, Switch1/2
  Switch2/1 -> "CIO-CTRxx "/2
  Switch1/1 -> "CIO-CTRxx "/1
  level/1 -> Mux/4
  Demux/4 -> "CIO-CTRxx "/6
  Demux/3 -> "CIO-CTRxx "/5
  Demux/2 -> "CIO-CTRxx "/4
  Demux/1 -> "CIO-CTRxx "/3
  Logical Operator1/1 -> Logical Operator/1
  Sum4/1 -> Abs/1
  Unit Delay2/1 -> Sum4/2
  Logical Operator/1 -> Data Type Conversion2/1
  Combinatorial  Logic/1 -> Logical Operator/2
  Relational Operator/1 -> Data Type Conversion1/1
  Relational Operator1/1 -> Data Type Conversion5/1
  1/relFreq2/1 -> Relational Operator1/2
  Product/1 -> Switch2/1, Switch1/3, Sum/1
  1/relFreq1/1 -> Relational Operator/2

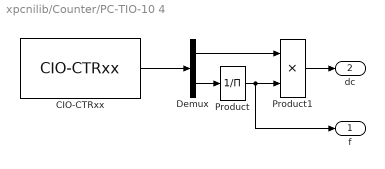
== system xpcnilib/Counter/PC-TIO-10 4 ==
  "CIO-CTRxx " : xpcmeasurementcomputinglib/Counter/CIO-CTRxx   mastermode=MasterMode  countermode=CounterMode  init=Init  commands=Runtime  term=Term  ts=Ts  baseAddress=baseAddress
  Demux : Demux  Outputs=2
  Product : Product  Inputs=/  SaturateOnIntegerOverflow=on  InputSameDT=on
  Product1 : Product  Inputs=**  SaturateOnIntegerOverflow=on  InputSameDT=on
  f : Outport
  dc : Outport  Port=2
  wires:
  Product1/1 -> dc/1
  Product/1 -> Product1/2, f/1
  Demux/2 -> Product/1
  Demux/1 -> Product1/1
  "CIO-CTRxx "/1 -> Demux/1

== system xpcnilib/Counter/PC-TIO-10 5 ==
  "CIO-CTRxx " : xpcmeasurementcomputinglib/Counter/CIO-CTRxx   mastermode=MasterMode  countermode=CounterMode  init=Init  commands=Runtime  term=Term  ts=Ts  baseAddress=baseAddress
  Product : Product  Inputs=/  SaturateOnIntegerOverflow=on  InputSameDT=on
  f : Outport
  wires:
  Product/1 -> f/1
  "CIO-CTRxx "/1 -> Product/1

== system xpcnilib/Digital Input/PC-TIO-10  ==
  DAC1 : S-Function  FunctionName=dinipctio10  Parameters=n_channels,port,sample_time,baseaddress
  out_1 : Outport  InitialOutput=0
  wires:
  DAC1/1 -> out_1/1

== system xpcnilib/Digital Output/PC-TIO-10  ==
  in_1 : Inport  LatchInput=off
  DAC : S-Function  FunctionName=donipctio10  Parameters=n_channels,port,sample_time,baseaddress
  wires:
  in_1/1 -> DAC/1
